simulink subsystem "Gearbox"  (R2022b)
settings: Solver=VariableStepAuto  StartTime=0.0  StopTime=10.0  RelTol=1e-3
model mask{i=10, J=10}
  mask prompts: i "Gear ratio"; J "Moment of inertia"
settings Model: Creator=Maxim Kozlov  LastModifiedBy=Maxim Kozlov
settings OptimizationCC: ReuseModelBlockBuffer=on

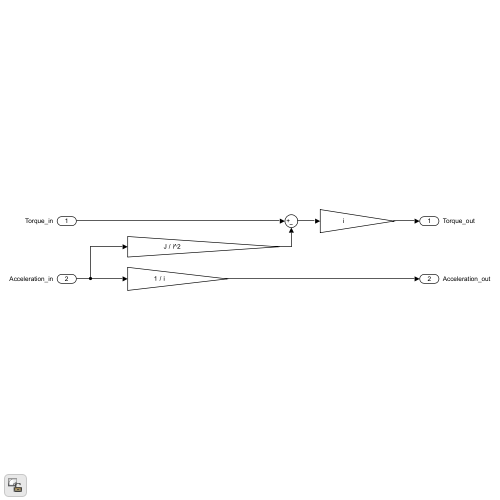
[thumbnail: Simulink's stored preview of the top-level diagram]
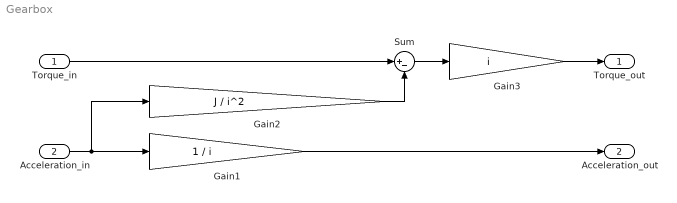
== system Gearbox ==
  Torque_in : Inport
  Acceleration_in : Inport  Port=2
  Gain1 : Gain  Gain=1 / i
  Gain2 : Gain  Gain=J / i^2
  Gain3 : Gain  Gain=i
  Sum : Sum  Inputs=|+-
  Torque_out : Outport
  Acceleration_out : Outport  Port=2
  wires:
  Acceleration_in/1 -> Gain1/1, Gain2/1
  Sum/1 -> Gain3/1
  Gain1/1 -> Acceleration_out/1
  Gain2/1 -> Sum/2
  Gain3/1 -> Torque_out/1
  Torque_in/1 -> Sum/1
